simulink model "mainSimulink_localPi"  (R2021a)
settings: Solver=VariableStepAuto  StartTime=0.0  StopTime=20  FixedStep=samplingTime  RelTol=1e-3
model workspace (MATLAB code in the model file):
  | %% Simulink settings
  | controllerFile = 'directFFcontroller';
  | set_param('mainSimulink_localPi/Subsystem Reference', 'ReferencedSubsystem', controllerFile);
  | %% Display settings
  | scopeTimeSpan = 30;
  | 
  | %% Robot settings (must match Python)
  | sensorFreq = 125;
  | actuatorFreq = 125;
  | TCPport = 12345;
  | dataSize = 2;
  | sensorSamplingTime = 1/sensorFreq;
  | actuatorTime = 1/actuatorFreq;
undefined symbols (not defined in the file): f
libraries: instrumentlib x2
settings Model: Creator=chukh  LastModifiedBy=chukh

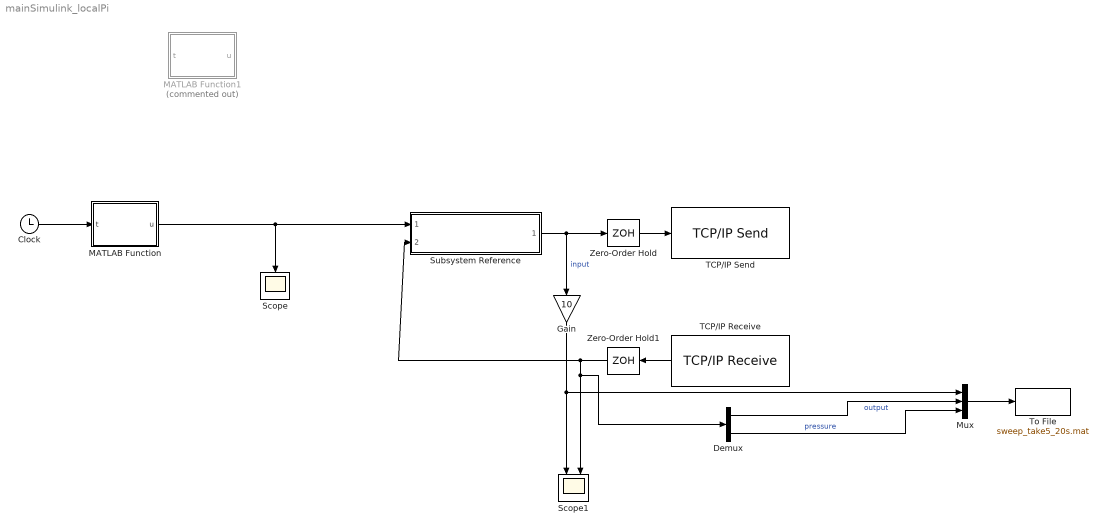
== system mainSimulink_localPi ==
  Clock : Clock
  Demux : Demux  Outputs=2
  Gain : Gain  Gain=10
  MATLAB Function : MATLAB Function  TreatAsAtomicUnit=on
  MATLAB Function1 : MATLAB Function  Commented=on  TreatAsAtomicUnit=on
  Mux : Mux  Inputs=3
  Scope : Scope
  Scope1 : Scope  NumInputPorts=2
  Subsystem Reference : Subsystem  ReferencedSubsystem=directFFcontroller
  TCP/IP Receive : instrumentlib/TCP//IP Receive  Host=server.softrobot  Port=TCPport  DataSize=dataSize  EnableBlockingMode=on  Timeout=0.5  SampleTime=sensorSamplingTime  DataType=double  ByteOrder=LittleEndian  ASCIIFormatting=%f,  Terminator=LF
  TCP/IP Send : instrumentlib/TCP//IP Send  Host=server.softrobot  Port=TCPport  EnableBlockingMode=on  Timeout=0.5  ByteOrder=LittleEndian  TransferDelay=on
  To File : ToFile  Filename=sweep_take5_20s.mat  MatrixName=data  SaveFormat=Timeseries
  Zero-Order Hold : ZeroOrderHold  SampleTime=actuatorTime
  Zero-Order Hold1 : ZeroOrderHold  SampleTime=actuatorTime
  wires:
  Subsystem Reference/1 -> Gain/1, Zero-Order Hold/1  "input"
  TCP/IP Receive/1 -> Zero-Order Hold1/1
  Zero-Order Hold/1 -> TCP/IP Send/1
  Zero-Order Hold1/1 -> Subsystem Reference/2, Demux/1, Scope1/2
  MATLAB Function/1(u) -> Scope/1, Subsystem Reference/1
  Demux/1 -> Mux/2  "output"
  Demux/2 -> Mux/3  "pressure"
  Mux/1 -> To File/1
  Clock/1 -> MATLAB Function/1(t)
  Gain/1 -> Scope1/1, Mux/1

== matlab function mainSimulink_localPi/MATLAB Function1 ==
  data: t input; u output
function u = sweepSignal(t)
u = 0.5+0.4*sin(0.25*t^2);

== matlab function mainSimulink_localPi/MATLAB Function ==
  data: t input; u output
function u = upAndDown(t)
period = 10;
u = 0.5+0.4*sin(0.25*t^2);
